simulink subsystem "parkinv"  (R2020a)
settings: Solver=VariableStepAuto  StartTime=0.0  StopTime=10.0  RelTol=1e-3
libraries: simulink x1
settings Model: Creator=ZhuanZ（无密码）  LastModifiedBy=ZhuanZ（无密码）

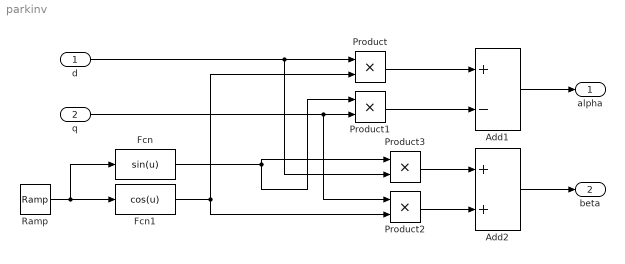
== system parkinv ==
  d : Inport
  q : Inport  Port=2
  Add1 : Sum  Inputs=+-
  Add2 : Sum
  Fcn : Fcn  Expr=sin(u)
  Fcn1 : Fcn  Expr=cos(u)
  Product{,1..3} (4 alike) : Product  RndMeth=Zero
  Ramp : simulink/Sources/Ramp  slope=1  start=0  InitialOutput=0
  alpha : Outport
  beta : Outport  Port=2
  wires:
  Product1/1 -> Add1/2
  Ramp/1 -> Fcn1/1, Fcn/1
  q/1 -> Product2/1, Product1/2
  Add2/1 -> beta/1
  Product2/1 -> Add2/2
  Product3/1 -> Add2/1
  Add1/1 -> alpha/1
  Fcn1/1 -> Product2/2, Product/2
  Fcn/1 -> Product1/1, Product3/1
  d/1 -> Product/1, Product3/2
  Product/1 -> Add1/1
